simulink model "transferfunction12A_Control"  (R2022b)
settings: Solver=VariableStepAuto  StartTime=t(1)  StopTime=t(end)  RelTol=1e-3
values from neighbouring files (symbols this model uses):
  EX4_SENS_DEN = [1]    [Analysis.m]
  EX4_SENS_NUM = [1]    [Analysis.m]
  T_DELAY = 0.006996183416    [Analysis.m]
settings Model: Creator=debber  LastModifiedBy=debber
settings DataIOCC: LoadExternalInput=on  SaveFormat=Array  OutputSaveName=y

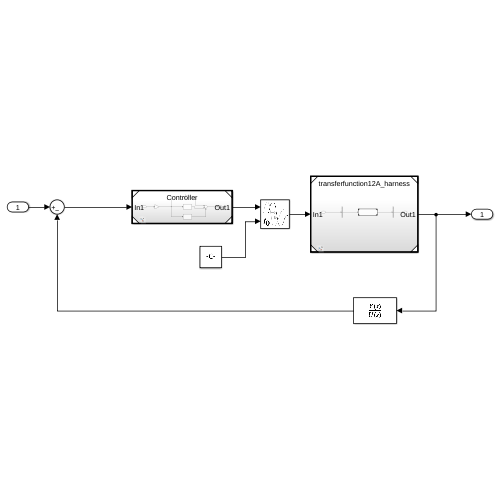
[thumbnail: Simulink's stored preview of the top-level diagram]
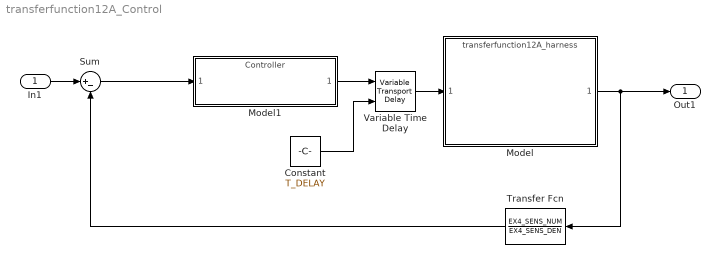
== system transferfunction12A_Control ==
  In1 : Inport
  Constant : Constant  Value=T_DELAY
  Model : ModelReference  ModelNameDialog=transferfunction12A_harness.slx  SimulationMode=Normal  ShowModelTerminatePort=on  ModelReferenceVersion=1.3
  Model1 : ModelReference  ModelNameDialog=Controller.slx  SimulationMode=Normal  ModelReferenceVersion=1.7
  Sum : Sum  Inputs=|+-
  Transfer Fcn : TransferFcn  Numerator=EX4_SENS_NUM  Denominator=EX4_SENS_DEN
  Variable Time Delay : VariableTransportDelay  MaximumDelay=10  ZeroDelay=on
  Out1 : Outport
  wires:
  In1/1 -> Sum/1
  Sum/1 -> Model1/1
  Transfer Fcn/1 -> Sum/2
  Model/1 -> Out1/1, Transfer Fcn/1
  Model1/1 -> Variable Time Delay/1
  Variable Time Delay/1 -> Model/1
  Constant/1 -> Variable Time Delay/2
